simulink model "ballbeam_sim"  (R2015a)
settings: Solver=ode45  StartTime=0.0  StopTime=200  RelTol=1e-3
InitFcn:
  | param
undefined symbols (not defined in the file or in its folder): ballbeam_ctrl, drawBallBeam, P
settings Model: Creator=beard  LastModifiedBy=beard
settings DataIOCC: SignalLoggingSaveFormat=ModelDataLogs
settings OptimizationCC: ExpressionDepthLimit=2147483647  InitFltsAndDblsToZero=on
settings DebuggingCC: UnderspecifiedInitializationDetection=Classic  MergeDetectMultiDrivingBlocksExec=none  SolverPrmCheckMsg=warning  FcnCallInpInsideContextMsg=UseLocalSettings  StateNameClashWarn=warning
settings GRTTargetCC: CombineOutputUpdateFcns=off  GRTInterface=on

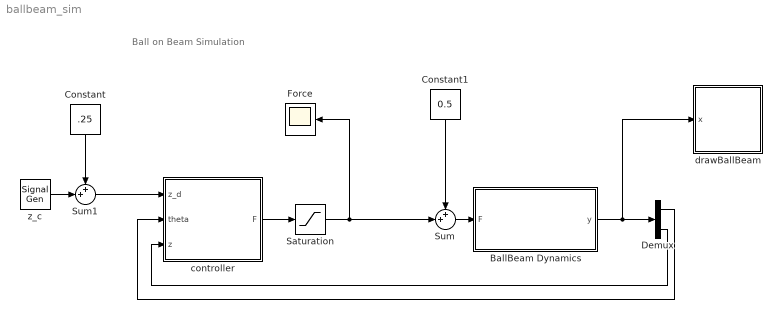
== system ballbeam_sim ==
  note: Ball on Beam Simulation
  BallBeam Dynamics : Subsystem
  Constant : Constant  Value=.25
  Constant1 : Constant  Value=0.5
  Demux : Demux  Outputs=2
  Force : Scope
      settings: YMin=-2.5  YMax=15  SaveName=ScopeData2
  Saturation : Saturate  UpperLimit=P.Fmax  LowerLimit=-P.Fmax
  Sum : Sum  Inputs=++|
  Sum1 : Sum  Inputs=++|
  controller : Subsystem
  drawBallBeam : Subsystem
      mask Display: image(imread('tv.jpg'))
  z_c : SignalGenerator  WaveForm=square  Amplitude=.15  Frequency=.02
  wires:
  z_c/1 -> Sum1/2
  Sum1/1 -> controller/1(z_d)
  Constant/1 -> Sum1/1
  controller/1(F) -> Saturation/1
  Demux/2 -> controller/3(z)
  Demux/1 -> controller/2(theta)
  Saturation/1 -> Sum/2, Force/1
  Sum/1 -> BallBeam Dynamics/1("F ")
  BallBeam Dynamics/1(y) -> drawBallBeam/1(x), Demux/1
  Constant1/1 -> Sum/1

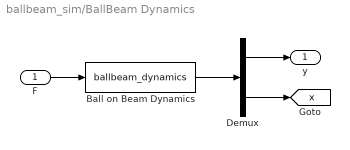
== system ballbeam_sim/BallBeam Dynamics ==
  "F " : Inport
  Ball on Beam Dynamics : S-Function  FunctionName=ballbeam_dynamics  Parameters=AP
  Demux : Demux  Outputs=[2;4]
  y : Outport
  tag scope: x=global
  wires:
  "F "/1 -> Ball on Beam Dynamics/1
  Ball on Beam Dynamics/1 -> Demux/1
  Demux/2 -> [x]
  Demux/1 -> y/1

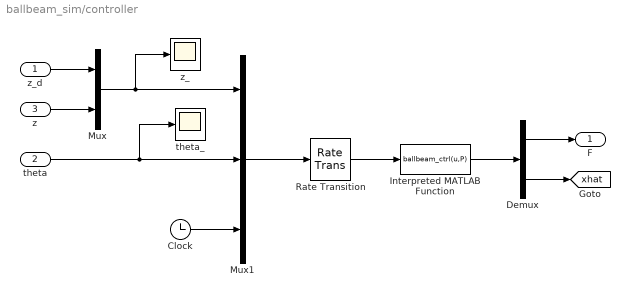
== system ballbeam_sim/controller ==
  z_d : Inport
  theta : Inport  Port=2
  z : Inport  Port=3
  Clock : Clock
  Demux : Demux  Outputs=[1;4]
  Interpreted MATLAB Function : MATLABFcn  MATLABFcn=ballbeam_ctrl(u,P)  OutputDimensions=1+4
  Mux : Mux  Inputs=2
  Mux1 : Mux  Inputs=3
  Rate Transition : RateTransition  OutPortSampleTime=P.Ts
  theta_ : Scope
      settings: TimeRange=100  YMin=-0.035  YMax=0.0125
  z_ : Scope
      settings: TimeRange=100  YMin=-0.05  YMax=0.425
  F : Outport
  tag scope: xhat=global
  wires:
  Mux1/1 -> Rate Transition/1
  Rate Transition/1 -> Interpreted MATLAB Function/1
  theta/1 -> theta_/1, Mux1/2
  z_d/1 -> Mux/1
  z/1 -> Mux/2
  Mux/1 -> z_/1, Mux1/1
  Clock/1 -> Mux1/3
  Interpreted MATLAB Function/1 -> Demux/1
  Demux/1 -> F/1
  Demux/2 -> [xhat]

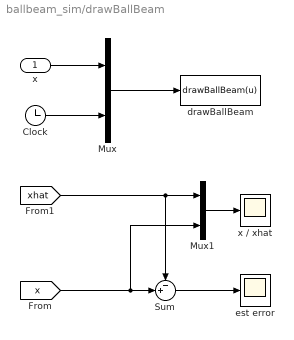
== system ballbeam_sim/drawBallBeam ==
  x : Inport
  Clock : Clock
  Mux : Mux  Inputs=2
  Mux1 : Mux  Inputs=2
  Sum : Sum  Inputs=-+|
  drawBallBeam : MATLABFcn  MATLABFcn=drawBallBeam(u)  OutputDimensions=0  SampleTime=0.1
  est error : Scope
      settings: TimeRange=40  YMin=-0.4  YMax=0.4  SaveName=ScopeData3
  x / xhat : Scope
      settings: TimeRange=40  YMin=-1.75  YMax=1.75  SaveName=ScopeData4
  wires:
  Mux/1 -> drawBallBeam/1
  x/1 -> Mux/1
  Clock/1 -> Mux/2
  Mux1/1 -> x / xhat/1
  Sum/1 -> est error/1
  [xhat] -> Mux1/1, Sum/1
  [x] -> Mux1/2, Sum/2
